simulink library "ControlAllocator"  (R2015b)
settings: Solver=VariableStepAuto  StartTime=0.0  StopTime=10.0  RelTol=1e-3
undefined symbols (not defined in the file or in its folder): SimIn
settings Model: Creator=cteubert  LastModifiedBy=cteubert

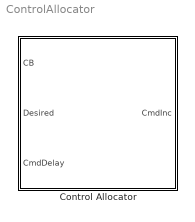
== system ControlAllocator ==
  Control Allocator : Subsystem  Variant=on

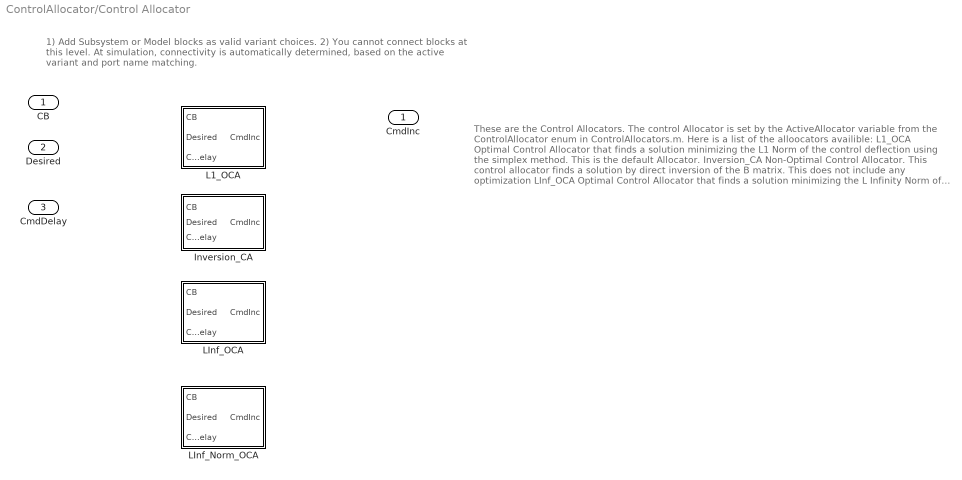
== system ControlAllocator/Control Allocator ==
  note: These are the Control Allocators. The control Allocator is set by the ActiveAllocator variable
      | from the ControlAllocator enum in ControlAllocators.m. Here is a list of the alloocators availible:
      |
      | L1_OCA
      | Optimal Control Allocator that finds a solution minimizing the L1 Norm of the control deflection using the simplex method. This is the default Allocator.
      |
      | Inversion_CA
      | Non-Optimal Control Allocator. This control allocator finds a solution by direct inversion of the B matrix. This does not include any optimization
      |
      | LInf_OCA
      | Optimal Control Allocator that finds a solution minimizing the L Infinity Norm of the control deflection using the simplex method.
      |
      | LInf_Norm_OCA
      | Optimal Control Allocator that finds a solution minimizing the normalized L Infinity Norm of the control deflection using the simplex method. [NOTE: This OCA is currently not functional]
  note: 1) Add Subsystem or Model blocks as valid variant choices.
      | 2) You cannot connect blocks at this level. At simulation, connectivity is automatically
      | determined, based on the active variant and port name matching.
  CB : Inport
  Desired : Inport  Port=2
  CmdDelay : Inport  Port=3
  Inversion_CA : Subsystem  VariantControl=ActiveAllocator==ControlAllocators.Inversion_CA
  L1_OCA : Subsystem  VariantControl=ActiveAllocator==ControlAllocators.L1_OCA
  LInf_Norm_OCA : Subsystem  VariantControl=ActiveAllocator==ControlAllocators.LInf_Norm_OCA
  LInf_OCA : Subsystem  VariantControl=ActiveAllocator==ControlAllocators.LInf_OCA
  CmdInc : Outport

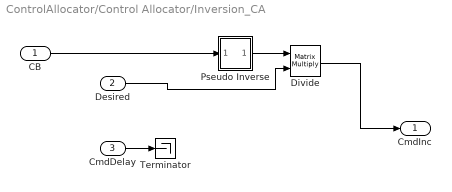
== system ControlAllocator/Control Allocator/Inversion_CA ==
  CB : Inport
  Desired : Inport  Port=2
  CmdDelay : Inport  Port=3
  Divide : Product  Multiplication=Matrix(*)
  Pseudo Inverse : Subsystem
  Terminator : Terminator
  CmdInc : Outport
  wires:
  CmdDelay/1 -> Terminator/1
  Pseudo Inverse/1(Out1) -> Divide/1
  CB/1 -> Pseudo Inverse/1(In1)
  Desired/1 -> Divide/2
  Divide/1 -> CmdInc/1

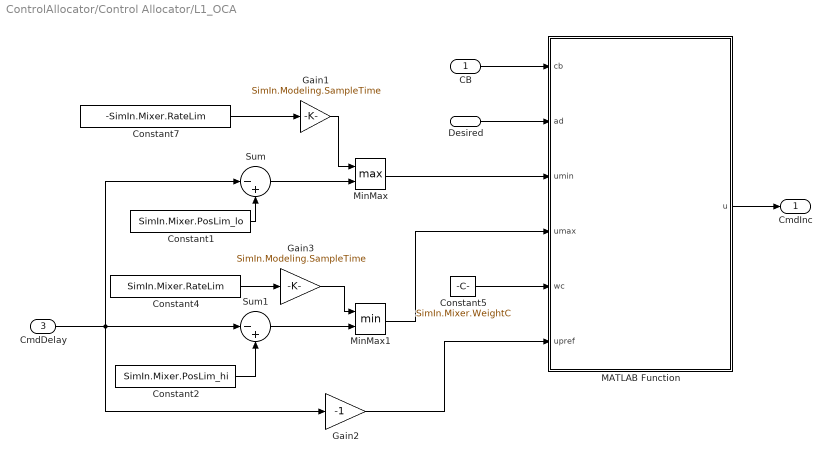
== system ControlAllocator/Control Allocator/L1_OCA ==
  CB : Inport
  Desired : Inport  Port=2
  CmdDelay : Inport  Port=3
  Constant1 : Constant  Value=SimIn.Mixer.PosLim_lo
  Constant2 : Constant  Value=SimIn.Mixer.PosLim_hi
  Constant4 : Constant  Value=SimIn.Mixer.RateLim
  Constant5 : Constant  Value=SimIn.Mixer.WeightC
  Constant7 : Constant  Value=-SimIn.Mixer.RateLim
  Gain1 : Gain  Gain=SimIn.Modeling.SampleTime
  Gain2 : Gain  Gain=-1
  Gain3 : Gain  Gain=SimIn.Modeling.SampleTime
  MATLAB Function : MATLAB Function  TreatAsAtomicUnit=on
  MinMax : MinMax  Function=max  Inputs=2
  MinMax1 : MinMax  Inputs=2
  Sum : Sum  Inputs=|-+
  Sum1 : Sum  Inputs=|-+
  CmdInc : Outport
  wires:
  Gain3/1 -> MinMax1/1
  Gain1/1 -> MinMax/1
  MinMax1/1 -> MATLAB Function/4(umax)
  MinMax/1 -> MATLAB Function/3(umin)
  Constant7/1 -> Gain1/1
  Constant4/1 -> Gain3/1
  CmdDelay/1 -> Sum1/1, Gain2/1, Sum/1
  Constant2/1 -> Sum1/2
  Sum1/1 -> MinMax1/2
  Constant1/1 -> Sum/2
  Sum/1 -> MinMax/2
  Gain2/1 -> MATLAB Function/6(upref)
  CB/1 -> MATLAB Function/1(cb)
  Desired/1 -> MATLAB Function/2(ad)
  Constant5/1 -> MATLAB Function/5(wc)
  MATLAB Function/1(u) -> CmdInc/1

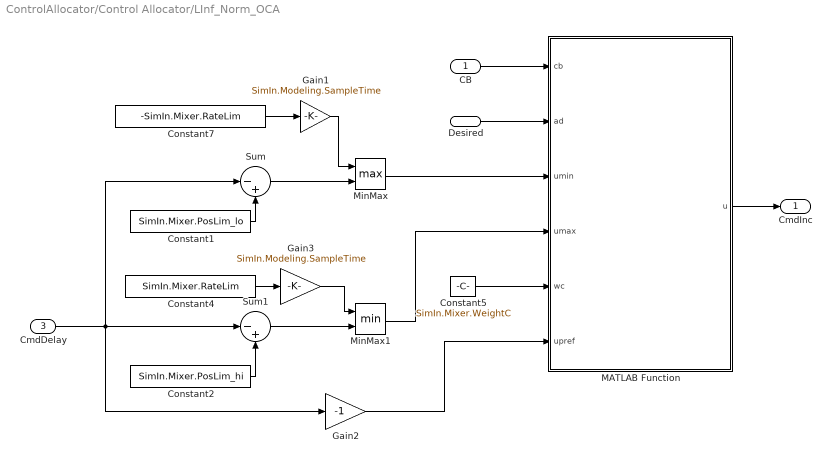
== system ControlAllocator/Control Allocator/LInf_Norm_OCA ==
  CB : Inport
  Desired : Inport  Port=2
  CmdDelay : Inport  Port=3
  Constant1 : Constant  Value=SimIn.Mixer.PosLim_lo
  Constant2 : Constant  Value=SimIn.Mixer.PosLim_hi
  Constant4 : Constant  Value=SimIn.Mixer.RateLim
  Constant5 : Constant  Value=SimIn.Mixer.WeightC
  Constant7 : Constant  Value=-SimIn.Mixer.RateLim
  Gain1 : Gain  Gain=SimIn.Modeling.SampleTime
  Gain2 : Gain  Gain=-1
  Gain3 : Gain  Gain=SimIn.Modeling.SampleTime
  MATLAB Function : MATLAB Function  TreatAsAtomicUnit=on
  MinMax : MinMax  Function=max  Inputs=2
  MinMax1 : MinMax  Inputs=2
  Sum : Sum  Inputs=|-+
  Sum1 : Sum  Inputs=|-+
  CmdInc : Outport
  wires:
  Gain3/1 -> MinMax1/1
  Gain1/1 -> MinMax/1
  MinMax1/1 -> MATLAB Function/4(umax)
  MinMax/1 -> MATLAB Function/3(umin)
  Constant7/1 -> Gain1/1
  Constant4/1 -> Gain3/1
  CmdDelay/1 -> Sum1/1, Gain2/1, Sum/1
  Constant2/1 -> Sum1/2
  Sum1/1 -> MinMax1/2
  Constant1/1 -> Sum/2
  Sum/1 -> MinMax/2
  Gain2/1 -> MATLAB Function/6(upref)
  CB/1 -> MATLAB Function/1(cb)
  Desired/1 -> MATLAB Function/2(ad)
  Constant5/1 -> MATLAB Function/5(wc)
  MATLAB Function/1(u) -> CmdInc/1

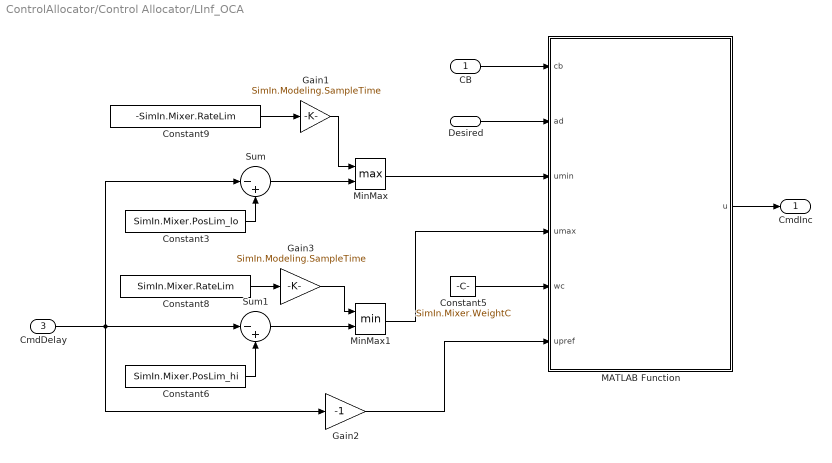
== system ControlAllocator/Control Allocator/LInf_OCA ==
  CB : Inport
  Desired : Inport  Port=2
  CmdDelay : Inport  Port=3
  Constant3 : Constant  Value=SimIn.Mixer.PosLim_lo
  Constant5 : Constant  Value=SimIn.Mixer.WeightC
  Constant6 : Constant  Value=SimIn.Mixer.PosLim_hi
  Constant8 : Constant  Value=SimIn.Mixer.RateLim
  Constant9 : Constant  Value=-SimIn.Mixer.RateLim
  Gain1 : Gain  Gain=SimIn.Modeling.SampleTime
  Gain2 : Gain  Gain=-1
  Gain3 : Gain  Gain=SimIn.Modeling.SampleTime
  MATLAB Function : MATLAB Function  TreatAsAtomicUnit=on
  MinMax : MinMax  Function=max  Inputs=2
  MinMax1 : MinMax  Inputs=2
  Sum : Sum  Inputs=|-+
  Sum1 : Sum  Inputs=|-+
  CmdInc : Outport
  wires:
  Gain3/1 -> MinMax1/1
  Gain1/1 -> MinMax/1
  MinMax1/1 -> MATLAB Function/4(umax)
  MinMax/1 -> MATLAB Function/3(umin)
  Constant9/1 -> Gain1/1
  Constant8/1 -> Gain3/1
  CmdDelay/1 -> Sum1/1, Gain2/1, Sum/1
  Constant6/1 -> Sum1/2
  Sum1/1 -> MinMax1/2
  Constant3/1 -> Sum/2
  Sum/1 -> MinMax/2
  Gain2/1 -> MATLAB Function/6(upref)
  CB/1 -> MATLAB Function/1(cb)
  Desired/1 -> MATLAB Function/2(ad)
  Constant5/1 -> MATLAB Function/5(wc)
  MATLAB Function/1(u) -> CmdInc/1

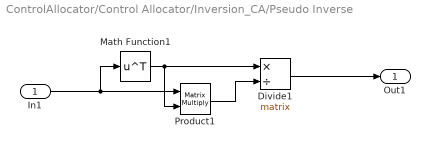
== system ControlAllocator/Control Allocator/Inversion_CA/Pseudo Inverse ==
  In1 : Inport
  Divide1 : Product  Inputs=*/  Multiplication=Matrix(*)
  Math Function1 : Math  Operator=transpose  SaturateOnIntegerOverflow=on
  Product1 : Product  Multiplication=Matrix(*)
  Out1 : Outport
  wires:
  Divide1/1 -> Out1/1
  Product1/1 -> Divide1/2
  In1/1 -> Product1/1, Math Function1/1
  Math Function1/1 -> Divide1/1, Product1/2

== matlab function ControlAllocator/Control Allocator/LInf_OCA/MATLAB Function ==
  data: u output; cb input; ad input; umin input; umax input; wc input; upref input
function u = runOCA(cb,ad,umin,umax,wc,upref)
%#codegen

[~, u] = LInf_OCA(cb,ad,umin,umax,wc,upref); % euinfx, euminx2

== matlab function ControlAllocator/Control Allocator/L1_OCA/MATLAB Function ==
  data: u output; cb input; ad input; umin input; umax input; wc input; upref input
function u = runOCA(cb,ad,umin,umax,wc,upref)
%#codegen

[~, u] = L1_OCA(cb,ad,umin,umax,wc,upref);

== matlab function ControlAllocator/Control Allocator/LInf_Norm_OCA/MATLAB Function ==
  data: u output; cb input; ad input; umin input; umax input; wc input; upref input
function u = runOCA(cb,ad,umin,umax,wc,upref)
%#codegen

[~, u] = LInf_Norm_OCA(cb,ad,umin,umax,wc,upref); % euinfx, euminx2
